simulink model "ALL_JP360_DBW_V6_5_1103"  (R2022a)
settings: Solver=FixedStepAuto  StartTime=0.0  StopTime=inf  FixedStep=0.01  RelTol=1e-3  EnableMultiTasking=on
model workspace (MAT data in the model file):
  g = 9.8
undefined symbols (not defined in the file or in its folder): canChannel, delta_v_p, IPM_Line_C0, IPM_Line_C1, IPM_Line_C2, IPM_Line_C3, M, M_p, MRR_ObjDistX, MRR_ObjDistY, MRR_ObjFusionCamID, MRR_ObjFusionSig, MRR_ObjID, MRR_ObjRelVelX, MRR_ObjRelVelY, MRR_ObjType, MRR_ObjUpdFlg, none, obj_vaild, untracktime, V, videoinput
libraries: canfdmsglib x230, canfdlib x76, slpidlib x24, simulink x18, dspstat3 x14, ctrlSharedLib x1, simulink_extras x1, imaqlib x1, realtime_pacer_lib x1, dspvision x1, visionsinks x1
(part 49 of 55)

== system ALL_JP360_DBW_V6_5_1103/MsgToCAN/CCAN_ADCU_MsgFromCAN/CCAN_ADCU_MRR_0x239 ==
  ACC_BrakePreferred : Inport
  ACC_Status : Inport  Port=2
  ACC_StandstillReq : Inport  Port=3
  ACC_DriveOff : Inport  Port=4
  Bus Creator : BusCreator  Inputs=16  OutDataTypeStr=Bus:CCAN_ADCU_MRR_0x239  NonVirtualBus=on
  Data Type Conversion{1,7,9,12,16} (5 alike) : DataTypeConversion  OutDataTypeStr=int8  SaturateOnIntegerOverflow=off  RndMeth=Floor
  Data Type Conversion{2..6,8,10,13,15} (9 alike) : DataTypeConversion  OutDataTypeStr=boolean  SaturateOnIntegerOverflow=off  RndMeth=Floor
  Data Type Conversion11 : DataTypeConversion  OutDataTypeStr=single  SaturateOnIntegerOverflow=off  RndMeth=Floor
  Data Type Conversion14 : DataTypeConversion  OutDataTypeStr=uint8  SaturateOnIntegerOverflow=off  RndMeth=Floor
  Rolling_Counter : simulink/User-Defined Functions/Rolling_Counter  SystemSampleTime=-1  VariantActivationTime=update diagram  Latency=0  AutoFrameSizeCalculation=off
      settings: SourceProductBaseCode=SL
  CCAN_ADCU_MRR_0x239FromOutData : Outport  OutDataTypeStr=Bus:CCAN_ADCU_MRR_0x239
  wires:
  Data Type Conversion1/1 -> Bus Creator/1  "ABA_Level"
  Data Type Conversion2/1 -> Bus Creator/2  "ABA_Req"
  Data Type Conversion3/1 -> Bus Creator/3  "ABP_Req"
  Data Type Conversion4/1 -> Bus Creator/4  "ACC_BrakePreferred"
  Data Type Conversion5/1 -> Bus Creator/5  "ACC_DriveOff"
  Data Type Conversion6/1 -> Bus Creator/6  "ACC_StandstillReq"
  Data Type Conversion7/1 -> Bus Creator/7  "ACC_Status"
  Data Type Conversion8/1 -> Bus Creator/8  "ACC_VLCMinBrakingReq"
  Data Type Conversion9/1 -> Bus Creator/9  "ACC_VLCShutdownMode"
  Data Type Conversion10/1 -> Bus Creator/10  "AEB_Req"
  Data Type Conversion11/1 -> Bus Creator/11  "AEB_TgtAx"
  Data Type Conversion12/1 -> Bus Creator/12  "AWB_Level"
  Data Type Conversion13/1 -> Bus Creator/13  "AWB_Req"
  Data Type Conversion14/1 -> Bus Creator/14  "Checksum_0x239"
  Data Type Conversion15/1 -> Bus Creator/15  "EBA_Req"
  Data Type Conversion16/1 -> Bus Creator/16  "RollingCounter_0x239"
  Bus Creator/1 -> CCAN_ADCU_MRR_0x239FromOutData/1  "CCAN_ADCU_MRR_0x239FromOutData"
  ACC_BrakePreferred/1 -> Data Type Conversion4/1
  ACC_StandstillReq/1 -> Data Type Conversion6/1
  ACC_Status/1 -> Data Type Conversion7/1
  Rolling_Counter/1 -> Data Type Conversion16/1
  ACC_DriveOff/1 -> Data Type Conversion5/1

== system ALL_JP360_DBW_V6_5_1103/MsgToCAN/CCAN_ADCU_MsgFromCAN/CCAN_ADCU_MRR_0x246 ==
  ACC_Status : Inport
  setvspped : Inport  Port=2
  ACC_TimeGapSet : Inport  Port=3
  ACC_EngineStartstop : Inport  Port=4
  Obj_Speed : Inport  Port=5
  ACC_ObjDetected : Inport  Port=6
  Bus Creator : BusCreator  Inputs=19  OutDataTypeStr=Bus:CCAN_ADCU_MRR_0x246  NonVirtualBus=on
  Constant : Constant  Value=2  OutDataTypeStr=int8
  Constant1 : Constant  Value=2  OutDataTypeStr=int8
  Constant2 : Constant  Value=2  OutDataTypeStr=int8
  Data Type Conversion{1,3,7..10,14..15,19} (9 alike) : DataTypeConversion  OutDataTypeStr=int8  SaturateOnIntegerOverflow=off  RndMeth=Floor
  Data Type Conversion11 : DataTypeConversion  OutDataTypeStr=uint8  SaturateOnIntegerOverflow=off  RndMeth=Floor
  Data Type Conversion{2,4,6,12..13,16..17} (7 alike) : DataTypeConversion  OutDataTypeStr=boolean  SaturateOnIntegerOverflow=off  RndMeth=Floor
  Data Type Conversion18 : DataTypeConversion  OutDataTypeStr=uint8  SaturateOnIntegerOverflow=off  RndMeth=Floor
  Data Type Conversion5 : DataTypeConversion  OutDataTypeStr=single  SaturateOnIntegerOverflow=off  RndMeth=Floor
  Rolling_Counter : simulink/User-Defined Functions/Rolling_Counter  SystemSampleTime=-1  VariantActivationTime=update diagram  Latency=0  AutoFrameSizeCalculation=off
      settings: SourceProductBaseCode=SL
  CCAN_ADCU_MRR_0x246FromOutData : Outport  OutDataTypeStr=Bus:CCAN_ADCU_MRR_0x246
  wires:
  Data Type Conversion1/1 -> Bus Creator/1  "ACC_EngineStartstop"
  Data Type Conversion2/1 -> Bus Creator/2  "ACC_FailInfo"
  Data Type Conversion3/1 -> Bus Creator/3  "ACC_ModeHMI"
  Data Type Conversion4/1 -> Bus Creator/4  "ACC_ObjDetected"
  Data Type Conversion5/1 -> Bus Creator/5  "ACC_SpdSetValue"
  Data Type Conversion6/1 -> Bus Creator/6  "ACC_TakeOverReq"
  Data Type Conversion7/1 -> Bus Creator/7  "ACC_TarObjBarDis"
  Data Type Conversion8/1 -> Bus Creator/8  "ACC_Textinfo"
  Data Type Conversion9/1 -> Bus Creator/9  "ACC_TimeGapSet"
  Data Type Conversion10/1 -> Bus Creator/10  "AEB_Status"
  Data Type Conversion11/1 -> Bus Creator/11  "Checksum_0x246"
  Data Type Conversion12/1 -> Bus Creator/12  "FCW_PedWarningLevel1"
  Data Type Conversion13/1 -> Bus Creator/13  "FCW_PedWarningLevel2"
  Data Type Conversion14/1 -> Bus Creator/14  "FCW_Sensitive"
  Data Type Conversion15/1 -> Bus Creator/15  "FCW_Status"
  Data Type Conversion16/1 -> Bus Creator/16  "FCW_WarningLevel1"
  Data Type Conversion17/1 -> Bus Creator/17  "FCW_WarningLevel2"
  Data Type Conversion18/1 -> Bus Creator/18  "Obj_Speed"
  Data Type Conversion19/1 -> Bus Creator/19  "RollingCounter_0x246"
  Bus Creator/1 -> CCAN_ADCU_MRR_0x246FromOutData/1  "CCAN_ADCU_MRR_0x246FromOutData"
  Rolling_Counter/1 -> Data Type Conversion19/1
  ACC_EngineStartstop/1 -> Data Type Conversion1/1
  ACC_Status/1 -> Data Type Conversion3/1
  setvspped/1 -> Data Type Conversion5/1
  ACC_TimeGapSet/1 -> Data Type Conversion9/1
  Constant/1 -> Data Type Conversion10/1
  Constant1/1 -> Data Type Conversion14/1
  Constant2/1 -> Data Type Conversion15/1
  Obj_Speed/1 -> Data Type Conversion18/1
  ACC_ObjDetected/1 -> Data Type Conversion4/1

== system ALL_JP360_DBW_V6_5_1103/MsgToCAN/CCAN_ADCU_MsgFromCAN/CCAN_ADCU_MRR_FRObj_0x279 ==
  MRR_F_Object_dx : Inport
  MRR_F_Object_dy : Inport  Port=2
  MRR_F_Obj_0x_class : Inport  Port=3
  Bus Creator : BusCreator  Inputs=8  OutDataTypeStr=Bus:CCAN_ADCU_MRR_FRObj_0x279  NonVirtualBus=on
  Data Type Conversion1 : DataTypeConversion  OutDataTypeStr=boolean  SaturateOnIntegerOverflow=off  RndMeth=Floor
  Data Type Conversion2 : DataTypeConversion  OutDataTypeStr=int8  SaturateOnIntegerOverflow=off  RndMeth=Floor
  Data Type Conversion{3..4,6..7} (4 alike) : DataTypeConversion  OutDataTypeStr=single  SaturateOnIntegerOverflow=off  RndMeth=Floor
  Data Type Conversion5 : DataTypeConversion  OutDataTypeStr=int8  SaturateOnIntegerOverflow=off  RndMeth=Floor
  Data Type Conversion8 : DataTypeConversion  OutDataTypeStr=boolean  SaturateOnIntegerOverflow=off  RndMeth=Floor
  CCAN_ADCU_MRR_FRObj_0x279FromOutData : Outport  OutDataTypeStr=Bus:CCAN_ADCU_MRR_FRObj_0x279
  wires:
  Data Type Conversion1/1 -> Bus Creator/1  "MRR_FFTargetDetection"
  Data Type Conversion2/1 -> Bus Creator/2  "MRR_FF_Obj_0x_class"
  Data Type Conversion3/1 -> Bus Creator/3  "MRR_FF_Object_dx"
  Data Type Conversion4/1 -> Bus Creator/4  "MRR_FF_Object_dy"
  Data Type Conversion5/1 -> Bus Creator/5  "MRR_F_Obj_0x_class"
  Data Type Conversion6/1 -> Bus Creator/6  "MRR_F_Object_dx"
  Data Type Conversion7/1 -> Bus Creator/7  "MRR_F_Object_dy"
  Data Type Conversion8/1 -> Bus Creator/8  "MRR_PedDetection"
  Bus Creator/1 -> CCAN_ADCU_MRR_FRObj_0x279FromOutData/1  "CCAN_ADCU_MRR_FRObj_0x279FromOutData"
  MRR_F_Object_dy/1 -> Data Type Conversion7/1
  MRR_F_Object_dx/1 -> Data Type Conversion6/1
  MRR_F_Obj_0x_class/1 -> Data Type Conversion5/1

== system ALL_JP360_DBW_V6_5_1103/MsgToCAN/CCAN_ADCU_MsgFromCAN/CCAN_ADCU_MRR_LRObj_0x480 ==
  MRR_L_Obj_0x_class : Inport
  MRR_L_Object_dx : Inport  Port=2
  MRR_L_Object_dy : Inport  Port=3
  MRR_LeftTargetDetection : Inport  Port=4
  MRR_R_Obj_0x_class : Inport  Port=5
  MRR_R_Object_dx : Inport  Port=6
  MRR_R_Object_dy : Inport  Port=7
  MRR_RightTargetDetection : Inport  Port=8
  Bus Creator : BusCreator  Inputs=8  OutDataTypeStr=Bus:CCAN_ADCU_MRR_LRObj_0x480  NonVirtualBus=on
  Data Type Conversion1 : DataTypeConversion  OutDataTypeStr=int8  SaturateOnIntegerOverflow=off  RndMeth=Floor
  Data Type Conversion{2..3,6..7} (4 alike) : DataTypeConversion  OutDataTypeStr=single  SaturateOnIntegerOverflow=off  RndMeth=Floor
  Data Type Conversion4 : DataTypeConversion  OutDataTypeStr=boolean  SaturateOnIntegerOverflow=off  RndMeth=Floor
  Data Type Conversion5 : DataTypeConversion  OutDataTypeStr=int8  SaturateOnIntegerOverflow=off  RndMeth=Floor
  Data Type Conversion8 : DataTypeConversion  OutDataTypeStr=boolean  SaturateOnIntegerOverflow=off  RndMeth=Floor
  CCAN_ADCU_MRR_LRObj_0x480FromOutData : Outport  OutDataTypeStr=Bus:CCAN_ADCU_MRR_LRObj_0x480
  wires:
  Data Type Conversion1/1 -> Bus Creator/1  "MRR_L_Obj_0x_class"
  Data Type Conversion2/1 -> Bus Creator/2  "MRR_L_Object_dx"
  Data Type Conversion3/1 -> Bus Creator/3  "MRR_L_Object_dy"
  Data Type Conversion4/1 -> Bus Creator/4  "MRR_LeftTargetDetection"
  Data Type Conversion5/1 -> Bus Creator/5  "MRR_R_Obj_0x_class"
  Data Type Conversion6/1 -> Bus Creator/6  "MRR_R_Object_dx"
  Data Type Conversion7/1 -> Bus Creator/7  "MRR_R_Object_dy"
  Data Type Conversion8/1 -> Bus Creator/8  "MRR_RightTargetDetection"
  Bus Creator/1 -> CCAN_ADCU_MRR_LRObj_0x480FromOutData/1  "CCAN_ADCU_MRR_LRObj_0x480FromOutData"
  MRR_L_Obj_0x_class/1 -> Data Type Conversion1/1
  MRR_L_Object_dx/1 -> Data Type Conversion2/1
  MRR_L_Object_dy/1 -> Data Type Conversion3/1
  MRR_LeftTargetDetection/1 -> Data Type Conversion4/1
  MRR_R_Obj_0x_class/1 -> Data Type Conversion5/1
  MRR_R_Object_dx/1 -> Data Type Conversion6/1
  MRR_R_Object_dy/1 -> Data Type Conversion7/1
  MRR_RightTargetDetection/1 -> Data Type Conversion8/1

== system ALL_JP360_DBW_V6_5_1103/MsgToCAN/CCAN_ADCU_MsgFromCAN/CCAN_ADCU_TIMESYNC_analy_620 ==
  Bus Creator : BusCreator  Inputs=6  OutDataTypeStr=Bus:CCAN_ADCU_TIMESYNC_analy_620  NonVirtualBus=on
  Data Type Conversion{1..5} (5 alike) : DataTypeConversion  OutDataTypeStr=int8  SaturateOnIntegerOverflow=off  RndMeth=Floor
  Data Type Conversion6 : DataTypeConversion  OutDataTypeStr=int16  SaturateOnIntegerOverflow=off  RndMeth=Floor
  CCAN_ADCU_TIMESYNC_analy_620FromOutData : Outport  OutDataTypeStr=Bus:CCAN_ADCU_TIMESYNC_analy_620
  wires:
  Data Type Conversion1/1 -> Bus Creator/1  "TIMESYNC_Date"
  Data Type Conversion2/1 -> Bus Creator/2  "TIMESYNC_Hour"
  Data Type Conversion3/1 -> Bus Creator/3  "TIMESYNC_Minute"
  Data Type Conversion4/1 -> Bus Creator/4  "TIMESYNC_Month"
  Data Type Conversion5/1 -> Bus Creator/5  "TIMESYNC_Second"
  Data Type Conversion6/1 -> Bus Creator/6  "TIMESYNC_Year"
  Bus Creator/1 -> CCAN_ADCU_TIMESYNC_analy_620FromOutData/1  "CCAN_ADCU_TIMESYNC_analy_620FromOutData"

== system ALL_JP360_DBW_V6_5_1103/MsgToCAN/CCAN_ADCU_MsgToCAN/CCAN_ADCU_ADCU_0x538 ==
  CCAN_ADCU_ADCU_0x538ToInData : Inport  OutDataTypeStr=Bus:CCAN_ADCU_ADCU_0x538
  CAN FD Pack : canfdmsglib/CAN FD Pack  CANdbFile=HiFire_JPT360_CCAN_Matrix_CAN_V1.72_VP_ADCU.dbc  MsgList=(none)  MsgName=ADCU_0x538  ProtocolMode=CAN FD  MsgIDType=Standard (11-bit identifier)  MsgIdentifier=1336  MsgLength=8  Remote=off  BRSSwitch=on  ApplyMinMax=off  SignalInfo={'ADCU_state','6','2','BE','unsigned','Standard','0','1','0','0','3';'BSD_FCTB_State','0','1','BE','unsigned','Standard','0','1','0','0','1'}
      settings: SourceProductBaseCode=XP,ME,VN  DataFormat=CANdb specified signals
  CAN FD Pack1 : BusSelector  OutputSignals=ADCU_state,BSD_FCTB_State
  CAN_FD_8bit_checksum : simulink/User-Defined Functions/CAN_FD_8bit_checksum  SystemSampleTime=-1  VariantActivationTime=update diagram  Latency=0  AutoFrameSizeCalculation=off
      settings: SourceProductBaseCode=SL
  CCAN_ADCU_ADCU_0x538ToOutData : Outport  OutDataTypeStr=Bus:CAN_FD_MESSAGE_BUS
  wires:
  CCAN_ADCU_ADCU_0x538ToInData/1 -> CAN FD Pack1/1  "CCAN_ADCU_ADCU_0x538ToInData"
  CAN FD Pack/1 -> CAN_FD_8bit_checksum/1  "CCAN_ADCU_ADCU_0x538ToOutData"
  CAN_FD_8bit_checksum/1 -> CCAN_ADCU_ADCU_0x538ToOutData/1  "CCAN_ADCU_ADCU_0x538ToOutData"
  CAN FD Pack1/1 -> CAN FD Pack/1  "<ADCU_state>"
  CAN FD Pack1/2 -> CAN FD Pack/2  "<BSD_FCTB_State>"

== system ALL_JP360_DBW_V6_5_1103/MsgToCAN/CCAN_ADCU_MsgToCAN/CCAN_ADCU_ADCU_CanTSyn_0x570 ==
  CCAN_ADCU_ADCU_CanTSyn_0x570ToInData : Inport  OutDataTypeStr=Bus:CCAN_ADCU_ADCU_CanTSyn_0x570
  CAN FD Pack : canfdmsglib/CAN FD Pack  CANdbFile=HiFire_JPT360_CCAN_Matrix_CAN_V1.72_VP_ADCU.dbc  MsgList=(none)  MsgName=ADCU_CanTSyn_0x570  ProtocolMode=CAN FD  MsgIDType=Standard (11-bit identifier)  MsgIdentifier=1392  MsgLength=8  Remote=off  BRSSwitch=on  ApplyMinMax=off  SignalInfo={'CanTSyn','56','64','BE','unsigned','Standard','0','1','0','0','1.84467440737095e+19'}
      settings: SourceProductBaseCode=XP,ME,VN  DataFormat=CANdb specified signals
  CAN FD Pack1 : BusSelector  OutputSignals=CanTSyn
  CAN_FD_8bit_checksum : simulink/User-Defined Functions/CAN_FD_8bit_checksum  SystemSampleTime=-1  VariantActivationTime=update diagram  Latency=0  AutoFrameSizeCalculation=off
      settings: SourceProductBaseCode=SL
  CCAN_ADCU_ADCU_CanTSyn_0x570ToOutData : Outport  OutDataTypeStr=Bus:CAN_FD_MESSAGE_BUS
  wires:
  CCAN_ADCU_ADCU_CanTSyn_0x570ToInData/1 -> CAN FD Pack1/1  "CCAN_ADCU_ADCU_CanTSyn_0x570ToInData"
  CAN FD Pack/1 -> CAN_FD_8bit_checksum/1  "CCAN_ADCU_ADCU_CanTSyn_0x570ToOutData"
  CAN_FD_8bit_checksum/1 -> CCAN_ADCU_ADCU_CanTSyn_0x570ToOutData/1  "CCAN_ADCU_ADCU_CanTSyn_0x570ToOutData"

== system ALL_JP360_DBW_V6_5_1103/MsgToCAN/CCAN_ADCU_MsgToCAN/CCAN_ADCU_ADCU_DiagResp ==
  CCAN_ADCU_ADCU_DiagRespToInData : Inport  OutDataTypeStr=Bus:CCAN_ADCU_ADCU_DiagResp
  CAN FD Pack : canfdmsglib/CAN FD Pack  CANdbFile=HiFire_JPT360_CCAN_Matrix_CAN_V1.72_VP_ADCU.dbc  MsgList=(none)  MsgName=ADCU_DiagResp  ProtocolMode=CAN FD  MsgIDType=Standard (11-bit identifier)  MsgIdentifier=1817  MsgLength=8  Remote=off  BRSSwitch=on  ApplyMinMax=off  SignalInfo={'DiagRespFromADCU','56','64','BE','unsigned','Standard','0','1','0','0','1.84467440737095e+19'}
      settings: SourceProductBaseCode=XP,ME,VN  DataFormat=CANdb specified signals
  CAN FD Pack1 : BusSelector  OutputSignals=DiagRespFromADCU
  CAN_FD_8bit_checksum : simulink/User-Defined Functions/CAN_FD_8bit_checksum  SystemSampleTime=-1  VariantActivationTime=update diagram  Latency=0  AutoFrameSizeCalculation=off
      settings: SourceProductBaseCode=SL
  CCAN_ADCU_ADCU_DiagRespToOutData : Outport  OutDataTypeStr=Bus:CAN_FD_MESSAGE_BUS
  wires:
  CCAN_ADCU_ADCU_DiagRespToInData/1 -> CAN FD Pack1/1  "CCAN_ADCU_ADCU_DiagRespToInData"
  CAN FD Pack/1 -> CAN_FD_8bit_checksum/1  "CCAN_ADCU_ADCU_DiagRespToOutData"
  CAN_FD_8bit_checksum/1 -> CCAN_ADCU_ADCU_DiagRespToOutData/1  "CCAN_ADCU_ADCU_DiagRespToOutData"

== system ALL_JP360_DBW_V6_5_1103/MsgToCAN/CCAN_ADCU_MsgToCAN/CCAN_ADCU_IPM_0x245 ==
  CCAN_ADCU_IPM_0x245ToInData : Inport  OutDataTypeStr=Bus:CCAN_ADCU_IPM_0x245
  CAN FD Pack : canfdmsglib/CAN FD Pack  CANdbFile=HiFire_JPT360_CCAN_Matrix_CAN_V1.72_VP_ADCU.dbc  MsgList=(none)  MsgName=IPM_0x245  ProtocolMode=CAN FD  MsgIDType=Standard (11-bit identifier)  MsgIdentifier=581  MsgLength=8  Remote=off  BRSSwitch=on  ApplyMinMax=off  SignalInfo={'Checksum_0x245','56','8','BE','unsigned','Standard','0','1','0','0','255';'IPM_ADAS_Alerts','43','3','BE','unsigned','Standard','0','1','0','0','7';'IPM_IHC_HighbeamReq','55','1','BE','unsigned','Standard','0','1','0','0','1';'IPM_IHC_Status','40','3','BE','unsigned','Standard','0','1','0','0','7';'IPM_LDWWarningType','52','2','BE','unsigned','Standard','0','1','0','0','3';'IPM_LaneAssitType','22','3','BE','unsigned','Standard','0','1','0','0','7';'IPM_LaneAssit_HandsonReq','54','1','BE','unsigned','Standard','0','1','0','0','1';'IPM_LaneAssit_LeftVisualization','18','2','BE','unsigned','Standard','0','1','0','0','3';'IPM_LaneAssit_RightVisualization','20','2','BE','unsigned','Standard','0','1','0','0','3';'IPM_LaneAssit_Sensitivity','16','1','BE','unsigned','Standard','0','1','0','0','1';'IPM_LaneAssit_Status','29','3','BE','unsigned','Standard','0','1','0','0','7';'IPM_LaneAssit_TorqueReq','13','11','BE','unsigned','Standard','0','0.01','-10.24','-10.24','10.22';'IPM_LaneAssit_TorqueReqStatus','10','2','BE','unsigned','Standard','0','1','0','0','3';'IPM_LaneAssit_TorqueValidity','12','1','BE','unsigned','Standard','0','1','0','0','1';'IPM_LaneAssit_WarningAudio','17','1','BE','unsigned','Standard','0','1','0','0','1';'IPM_LaneAssit_WarningVibration','9','1','BE','unsigned','Standard','0','1','0','0','1';'IPM_SLA_Spdlimit','32','8','BE','unsigned','Standard','0','1','0','0','255';'IPM_SLA_SpdlimitUnits','24','2','BE','unsigned','Standard','0','1','0','0','3';'IPM_SLA_Status','26','3','BE','unsigned','Standard','0','1','0','0','7';'IPM_TJAICA_Status','47','1','BE','unsigned','Standard','0','1','0','0','1';'RollingCounter_0x245','48','4','BE','unsigned','Standard','0','1','0','0','15'}
      settings: SourceProductBaseCode=XP,ME,VN  DataFormat=CANdb specified signals
  CAN FD Pack1 : BusSelector  OutputSignals=Checksum_0x245,IPM_ADAS_Alerts,IPM_IHC_HighbeamReq,IPM_IHC_Status,IPM_LDWWarningType,IPM_LaneAssitType,IPM_LaneAssit_HandsonReq,IPM_LaneAssit_LeftVisualization,IPM_LaneAssit_RightVisualization,IPM_LaneAssit_Sensitivity,IPM_LaneAssit_Status,IPM_LaneAssit_TorqueReq,IPM_LaneAssit_TorqueReqStatus,IPM_LaneAssit_TorqueValidity,IPM_LaneAssit_WarningAudio,IPM_LaneAssit_WarningVibration,IPM_SLA_Spdlimit,IPM_SLA_SpdlimitUnits,IPM_SLA_Status,IPM_TJAICA_Status,RollingCounter_0x245
  CAN_FD_8bit_checksum : simulink/User-Defined Functions/CAN_FD_8bit_checksum  SystemSampleTime=-1  VariantActivationTime=update diagram  Latency=0  AutoFrameSizeCalculation=off
      settings: SourceProductBaseCode=SL
  CCAN_ADCU_IPM_0x245ToOutData : Outport  OutDataTypeStr=Bus:CAN_FD_MESSAGE_BUS
  wires:
  CCAN_ADCU_IPM_0x245ToInData/1 -> CAN FD Pack1/1  "CCAN_ADCU_IPM_0x245ToInData"
  CAN FD Pack/1 -> CAN_FD_8bit_checksum/1  "CCAN_ADCU_IPM_0x245ToOutData"
  CAN_FD_8bit_checksum/1 -> CCAN_ADCU_IPM_0x245ToOutData/1  "CCAN_ADCU_IPM_0x245ToOutData"
  CAN FD Pack1/1 -> CAN FD Pack/1  "<Checksum_0x245>"
  CAN FD Pack1/2 -> CAN FD Pack/2  "<IPM_ADAS_Alerts>"
  CAN FD Pack1/3 -> CAN FD Pack/3  "<IPM_IHC_HighbeamReq>"
  CAN FD Pack1/4 -> CAN FD Pack/4  "<IPM_IHC_Status>"
  CAN FD Pack1/5 -> CAN FD Pack/5  "<IPM_LDWWarningType>"
  CAN FD Pack1/6 -> CAN FD Pack/6  "<IPM_LaneAssitType>"
  CAN FD Pack1/7 -> CAN FD Pack/7  "<IPM_LaneAssit_HandsonReq>"
  CAN FD Pack1/8 -> CAN FD Pack/8  "<IPM_LaneAssit_LeftVisualization>"
  CAN FD Pack1/9 -> CAN FD Pack/9  "<IPM_LaneAssit_RightVisualization>"
  CAN FD Pack1/10 -> CAN FD Pack/10  "<IPM_LaneAssit_Sensitivity>"
  CAN FD Pack1/11 -> CAN FD Pack/11  "<IPM_LaneAssit_Status>"
  CAN FD Pack1/12 -> CAN FD Pack/12  "<IPM_LaneAssit_TorqueReq>"
  CAN FD Pack1/13 -> CAN FD Pack/13  "<IPM_LaneAssit_TorqueReqStatus>"
  CAN FD Pack1/14 -> CAN FD Pack/14  "<IPM_LaneAssit_TorqueValidity>"
  CAN FD Pack1/15 -> CAN FD Pack/15  "<IPM_LaneAssit_WarningAudio>"
  CAN FD Pack1/16 -> CAN FD Pack/16  "<IPM_LaneAssit_WarningVibration>"
  CAN FD Pack1/17 -> CAN FD Pack/17  "<IPM_SLA_Spdlimit>"
  CAN FD Pack1/18 -> CAN FD Pack/18  "<IPM_SLA_SpdlimitUnits>"
  CAN FD Pack1/19 -> CAN FD Pack/19  "<IPM_SLA_Status>"
  CAN FD Pack1/20 -> CAN FD Pack/20  "<IPM_TJAICA_Status>"
  CAN FD Pack1/21 -> CAN FD Pack/21  "<RollingCounter_0x245>"

== system ALL_JP360_DBW_V6_5_1103/MsgToCAN/CCAN_ADCU_MsgToCAN/CCAN_ADCU_IPM_0x247 ==
  CCAN_ADCU_IPM_0x247ToInData : Inport  OutDataTypeStr=Bus:CCAN_ADCU_IPM_0x247
  CAN FD Pack : canfdmsglib/CAN FD Pack  CANdbFile=HiFire_JPT360_CCAN_Matrix_CAN_V1.72_VP_ADCU.dbc  MsgList=(none)  MsgName=IPM_0x247  ProtocolMode=CAN FD  MsgIDType=Standard (11-bit identifier)  MsgIdentifier=583  MsgLength=8  Remote=off  BRSSwitch=on  ApplyMinMax=off  SignalInfo={'Checksum_0x247','56','8','BE','unsigned','Standard','0','1','0','0','255';'IPM_DCLCSts','5','3','BE','unsigned','Standard','0','1','0','0','7';'IPM_DCLC_manualfeedback','14','4','BE','unsigned','Standard','0','1','0','0','15';'IPM_ELKSts','2','3','BE','unsigned','Standard','0','1','0','0','7';'IPM_Traffic_Sign_Dis','16','8','BE','unsigned','Standard','0','1','0','0','255';'IPM_TurnIndicatorReq','12','2','BE','unsigned','Standard','0','1','0','0','3';'RollingCounter_0x247','48','4','BE','unsigned','Standard','0','1','0','0','15'}
      settings: SourceProductBaseCode=XP,ME,VN  DataFormat=CANdb specified signals
  CAN FD Pack1 : BusSelector  OutputSignals=Checksum_0x247,IPM_DCLCSts,IPM_DCLC_manualfeedback,IPM_ELKSts,IPM_Traffic_Sign_Dis,IPM_TurnIndicatorReq,RollingCounter_0x247
  CAN_FD_8bit_checksum : simulink/User-Defined Functions/CAN_FD_8bit_checksum  SystemSampleTime=-1  VariantActivationTime=update diagram  Latency=0  AutoFrameSizeCalculation=off
      settings: SourceProductBaseCode=SL
  CCAN_ADCU_IPM_0x247ToOutData : Outport  OutDataTypeStr=Bus:CAN_FD_MESSAGE_BUS
  wires:
  CCAN_ADCU_IPM_0x247ToInData/1 -> CAN FD Pack1/1  "CCAN_ADCU_IPM_0x247ToInData"
  CAN FD Pack/1 -> CAN_FD_8bit_checksum/1  "CCAN_ADCU_IPM_0x247ToOutData"
  CAN_FD_8bit_checksum/1 -> CCAN_ADCU_IPM_0x247ToOutData/1  "CCAN_ADCU_IPM_0x247ToOutData"
  CAN FD Pack1/1 -> CAN FD Pack/1  "<Checksum_0x247>"
  CAN FD Pack1/2 -> CAN FD Pack/2  "<IPM_DCLCSts>"
  CAN FD Pack1/3 -> CAN FD Pack/3  "<IPM_DCLC_manualfeedback>"
  CAN FD Pack1/4 -> CAN FD Pack/4  "<IPM_ELKSts>"
  CAN FD Pack1/5 -> CAN FD Pack/5  "<IPM_Traffic_Sign_Dis>"
  CAN FD Pack1/6 -> CAN FD Pack/6  "<IPM_TurnIndicatorReq>"
  CAN FD Pack1/7 -> CAN FD Pack/7  "<RollingCounter_0x247>"

== system ALL_JP360_DBW_V6_5_1103/MsgToCAN/CCAN_ADCU_MsgToCAN/CCAN_ADCU_IPM_LeftLine_0x278 ==
  CCAN_ADCU_IPM_LeftLine_0x278ToInData : Inport  OutDataTypeStr=Bus:CCAN_ADCU_IPM_LeftLine_0x278
  CAN FD Pack : canfdmsglib/CAN FD Pack  CANdbFile=HiFire_JPT360_CCAN_Matrix_CAN_V1.72_VP_ADCU.dbc  MsgList=(none)  MsgName=IPM_LeftLine_0x278  ProtocolMode=CAN FD  MsgIDType=Standard (11-bit identifier)  MsgIdentifier=632  MsgLength=8  Remote=off  BRSSwitch=on  ApplyMinMax=off  SignalInfo={'IPM_LedtLine_dx_start','0','8','BE','unsigned','Standard','0','0.25','0','0','63.75';'IPM_LeftLine_dx_lookhead','27','9','BE','unsigned','Standard','0','0.25','0','0','127.75';'IPM_LeftLine_dy','20','12','BE','unsigned','Standard','0','0.0039062','-8','-8','7.9961';'IPM_LeftLine_hor_curvature_alteration','58','10','BE','unsigned','Standard','0','0.0001','-0.015','-0.015','0.0873';'IPM_LeftLine_hor_curve','33','10','BE','unsigned','Standard','0','0.0001','-0.015','-0.015','0.0873';'IPM_LeftLine_yawangle','52','12','BE','unsigned','Standard','0','0.00048828','-1','-1','0.99951'}
      settings: SourceProductBaseCode=XP,ME,VN  DataFormat=CANdb specified signals
  CAN FD Pack1 : BusSelector  OutputSignals=IPM_LedtLine_dx_start,IPM_LeftLine_dx_lookhead,IPM_LeftLine_dy,IPM_LeftLine_hor_curvature_alteration,IPM_LeftLine_hor_curve,IPM_LeftLine_yawangle
  CCAN_ADCU_IPM_LeftLine_0x278ToOutData : Outport  OutDataTypeStr=Bus:CAN_FD_MESSAGE_BUS
  wires:
  CCAN_ADCU_IPM_LeftLine_0x278ToInData/1 -> CAN FD Pack1/1  "CCAN_ADCU_IPM_LeftLine_0x278ToInData"
  CAN FD Pack/1 -> CCAN_ADCU_IPM_LeftLine_0x278ToOutData/1  "CCAN_ADCU_IPM_LeftLine_0x278ToOutData"
  CAN FD Pack1/1 -> CAN FD Pack/1  "<IPM_LedtLine_dx_start>"
  CAN FD Pack1/2 -> CAN FD Pack/2  "<IPM_LeftLine_dx_lookhead>"
  CAN FD Pack1/3 -> CAN FD Pack/3  "<IPM_LeftLine_dy>"
  CAN FD Pack1/4 -> CAN FD Pack/4  "<IPM_LeftLine_hor_curvature_alteration>"
  CAN FD Pack1/5 -> CAN FD Pack/5  "<IPM_LeftLine_hor_curve>"
  CAN FD Pack1/6 -> CAN FD Pack/6  "<IPM_LeftLine_yawangle>"

== system ALL_JP360_DBW_V6_5_1103/MsgToCAN/CCAN_ADCU_MsgToCAN/CCAN_ADCU_IPM_LeftLine_0x280 ==
  CCAN_ADCU_IPM_LeftLine_0x280ToInData : Inport  OutDataTypeStr=Bus:CCAN_ADCU_IPM_LeftLine_0x280
  CAN FD Pack : canfdmsglib/CAN FD Pack  CANdbFile=HiFire_JPT360_CCAN_Matrix_CAN_V1.72_VP_ADCU.dbc  MsgList=(none)  MsgName=IPM_LeftLine_0x280  ProtocolMode=CAN FD  MsgIDType=Standard (11-bit identifier)  MsgIdentifier=640  MsgLength=8  Remote=off  BRSSwitch=on  ApplyMinMax=off  SignalInfo={'IPM_LaneAssit_LeftLeftVisualization','0','2','BE','unsigned','Standard','0','1','0','0','3';'IPM_LeftLeftLine_Color','13','3','BE','unsigned','Standard','0','1','0','0','7';'IPM_LeftLeftLine_Type','10','3','BE','unsigned','Standard','0','1','0','0','7';'IPM_LeftLeftLine_curvature_alteration','56','12','BE','unsigned','Standard','0','0.0001','-0.015','-0.015','0.0873';'IPM_LeftLeftLine_dy','28','12','BE','unsigned','Standard','0','0.0039062','-8','-8','7.9961';'IPM_LeftLeftLine_hor_curve','33','10','BE','unsigned','Standard','0','0.0001','-0.015','-0.015','0.0873';'IPM_LeftLeftLine_yawangle','52','12','BE','unsigned','Standard','0','0.00048828','-1','-1','0.99951';'IPM_LeftLine_Color','5','3','BE','unsigned','Standard','0','1','0','0','7';'IPM_LeftLine_Type','2','3','BE','unsigned','Standard','0','1','0','0','7'}
      settings: SourceProductBaseCode=XP,ME,VN  DataFormat=CANdb specified signals
  CAN FD Pack1 : BusSelector  OutputSignals=IPM_LaneAssit_LeftLeftVisualization,IPM_LeftLeftLine_Color,IPM_LeftLeftLine_Type,IPM_LeftLeftLine_curvature_alteration,IPM_LeftLeftLine_dy,IPM_LeftLeftLine_hor_curve,IPM_LeftLeftLine_yawangle,IPM_LeftLine_Color,IPM_LeftLine_Type
  CCAN_ADCU_IPM_LeftLine_0x280ToOutData : Outport  OutDataTypeStr=Bus:CAN_FD_MESSAGE_BUS
  wires:
  CCAN_ADCU_IPM_LeftLine_0x280ToInData/1 -> CAN FD Pack1/1  "CCAN_ADCU_IPM_LeftLine_0x280ToInData"
  CAN FD Pack/1 -> CCAN_ADCU_IPM_LeftLine_0x280ToOutData/1  "CCAN_ADCU_IPM_LeftLine_0x280ToOutData"
  CAN FD Pack1/1 -> CAN FD Pack/1  "<IPM_LaneAssit_LeftLeftVisualization>"
  CAN FD Pack1/2 -> CAN FD Pack/2  "<IPM_LeftLeftLine_Color>"
  CAN FD Pack1/3 -> CAN FD Pack/3  "<IPM_LeftLeftLine_Type>"
  CAN FD Pack1/4 -> CAN FD Pack/4  "<IPM_LeftLeftLine_curvature_alteration>"
  CAN FD Pack1/5 -> CAN FD Pack/5  "<IPM_LeftLeftLine_dy>"
  CAN FD Pack1/6 -> CAN FD Pack/6  "<IPM_LeftLeftLine_hor_curve>"
  CAN FD Pack1/7 -> CAN FD Pack/7  "<IPM_LeftLeftLine_yawangle>"
  CAN FD Pack1/8 -> CAN FD Pack/8  "<IPM_LeftLine_Color>"
  CAN FD Pack1/9 -> CAN FD Pack/9  "<IPM_LeftLine_Type>"

== system ALL_JP360_DBW_V6_5_1103/MsgToCAN/CCAN_ADCU_MsgToCAN/CCAN_ADCU_IPM_RightLine_0x490 ==
  CCAN_ADCU_IPM_RightLine_0x490ToInData : Inport  OutDataTypeStr=Bus:CCAN_ADCU_IPM_RightLine_0x490
  CAN FD Pack : canfdmsglib/CAN FD Pack  CANdbFile=HiFire_JPT360_CCAN_Matrix_CAN_V1.72_VP_ADCU.dbc  MsgList=(none)  MsgName=IPM_RightLine_0x490  ProtocolMode=CAN FD  MsgIDType=Standard (11-bit identifier)  MsgIdentifier=1168  MsgLength=8  Remote=off  BRSSwitch=on  ApplyMinMax=off  SignalInfo={'IPM_RightLine_dx_lookhead','27','9','BE','unsigned','Standard','0','0.25','0','0','127.75';'IPM_RightLine_dx_start','0','8','BE','unsigned','Standard','0','0.25','0','0','63.75';'IPM_RightLine_dy','20','12','BE','unsigned','Standard','0','0.0039062','-8','-8','7.9961';'IPM_RightLine_hor_curvature_alteration','58','10','BE','unsigned','Standard','0','0.0001','-0.015','-0.015','0.0873';'IPM_RightLine_hor_curve','33','10','BE','unsigned','Standard','0','0.0001','-0.015','-0.015','0.0873';'IPM_RightLine_yawangle','52','12','BE','unsigned','Standard','0','0.00048828','-1','-1','0.99951'}
      settings: SourceProductBaseCode=XP,ME,VN  DataFormat=CANdb specified signals
  CAN FD Pack1 : BusSelector  OutputSignals=IPM_RightLine_dx_lookhead,IPM_RightLine_dx_start,IPM_RightLine_dy,IPM_RightLine_hor_curvature_alteration,IPM_RightLine_hor_curve,IPM_RightLine_yawangle
  CCAN_ADCU_IPM_RightLine_0x490ToOutData : Outport  OutDataTypeStr=Bus:CAN_FD_MESSAGE_BUS
  wires:
  CCAN_ADCU_IPM_RightLine_0x490ToInData/1 -> CAN FD Pack1/1  "CCAN_ADCU_IPM_RightLine_0x490ToInData"
  CAN FD Pack/1 -> CCAN_ADCU_IPM_RightLine_0x490ToOutData/1  "CCAN_ADCU_IPM_RightLine_0x490ToOutData"
  CAN FD Pack1/1 -> CAN FD Pack/1  "<IPM_RightLine_dx_lookhead>"
  CAN FD Pack1/2 -> CAN FD Pack/2  "<IPM_RightLine_dx_start>"
  CAN FD Pack1/3 -> CAN FD Pack/3  "<IPM_RightLine_dy>"
  CAN FD Pack1/4 -> CAN FD Pack/4  "<IPM_RightLine_hor_curvature_alteration>"
  CAN FD Pack1/5 -> CAN FD Pack/5  "<IPM_RightLine_hor_curve>"
  CAN FD Pack1/6 -> CAN FD Pack/6  "<IPM_RightLine_yawangle>"

== system ALL_JP360_DBW_V6_5_1103/MsgToCAN/CCAN_ADCU_MsgToCAN/CCAN_ADCU_IPM_RightLine_0x491 ==
  CCAN_ADCU_IPM_RightLine_0x491ToInData : Inport  OutDataTypeStr=Bus:CCAN_ADCU_IPM_RightLine_0x491
  CAN FD Pack : canfdmsglib/CAN FD Pack  CANdbFile=HiFire_JPT360_CCAN_Matrix_CAN_V1.72_VP_ADCU.dbc  MsgList=(none)  MsgName=IPM_RightLine_0x491  ProtocolMode=CAN FD  MsgIDType=Standard (11-bit identifier)  MsgIdentifier=1169  MsgLength=8  Remote=off  BRSSwitch=on  ApplyMinMax=off  SignalInfo={'IPM_LaneAssit_RightRightVisualization','0','2','BE','unsigned','Standard','0','1','0','0','3';'IPM_RighRightLine_Color','13','3','BE','unsigned','Standard','0','1','0','0','7';'IPM_RightLine_Color','5','3','BE','unsigned','Standard','0','1','0','0','7';'IPM_RightLine_Type','2','3','BE','unsigned','Standard','0','1','0','0','7';'IPM_RightRighLine_Type','10','3','BE','unsigned','Standard','0','1','0','0','7';'IPM_RightRightLine_curvature_alteration','56','12','BE','unsigned','Standard','0','0.0001','-0.015','-0.015','0.0873';'IPM_RightRightLine_dy','28','12','BE','unsigned','Standard','0','0.0039062','-8','-8','7.9961';'IPM_RightRightLine_hor_curve','33','10','BE','unsigned','Standard','0','0.0001','-0.015','-0.015','0.0873';'IPM_RightRightLine_yawangle','52','12','BE','unsigned','Standard','0','0.00048828','-1','-1','0.99951'}
      settings: SourceProductBaseCode=XP,ME,VN  DataFormat=CANdb specified signals
  CAN FD Pack1 : BusSelector  OutputSignals=IPM_LaneAssit_RightRightVisualization,IPM_RighRightLine_Color,IPM_RightLine_Color,IPM_RightLine_Type,IPM_RightRighLine_Type,IPM_RightRightLine_curvature_alteration,IPM_RightRightLine_dy,IPM_RightRightLine_hor_curve,IPM_RightRightLine_yawangle
  CCAN_ADCU_IPM_RightLine_0x491ToOutData : Outport  OutDataTypeStr=Bus:CAN_FD_MESSAGE_BUS
  wires:
  CCAN_ADCU_IPM_RightLine_0x491ToInData/1 -> CAN FD Pack1/1  "CCAN_ADCU_IPM_RightLine_0x491ToInData"
  CAN FD Pack/1 -> CCAN_ADCU_IPM_RightLine_0x491ToOutData/1  "CCAN_ADCU_IPM_RightLine_0x491ToOutData"
  CAN FD Pack1/1 -> CAN FD Pack/1  "<IPM_LaneAssit_RightRightVisualization>"
  CAN FD Pack1/2 -> CAN FD Pack/2  "<IPM_RighRightLine_Color>"
  CAN FD Pack1/3 -> CAN FD Pack/3  "<IPM_RightLine_Color>"
  CAN FD Pack1/4 -> CAN FD Pack/4  "<IPM_RightLine_Type>"
  CAN FD Pack1/5 -> CAN FD Pack/5  "<IPM_RightRighLine_Type>"
  CAN FD Pack1/6 -> CAN FD Pack/6  "<IPM_RightRightLine_curvature_alteration>"
  CAN FD Pack1/7 -> CAN FD Pack/7  "<IPM_RightRightLine_dy>"
  CAN FD Pack1/8 -> CAN FD Pack/8  "<IPM_RightRightLine_hor_curve>"
  CAN FD Pack1/9 -> CAN FD Pack/9  "<IPM_RightRightLine_yawangle>"

== system ALL_JP360_DBW_V6_5_1103/MsgToCAN/CCAN_ADCU_MsgToCAN/CCAN_ADCU_IPM_VLC_0x293 ==
  CCAN_ADCU_IPM_VLC_0x293ToInData : Inport  OutDataTypeStr=Bus:CCAN_ADCU_IPM_VLC_0x293
  CAN FD Pack : canfdmsglib/CAN FD Pack  CANdbFile=HiFire_JPT360_CCAN_Matrix_CAN_V1.72_VP_ADCU.dbc  MsgList=(none)  MsgName=IPM_VLC_0x293  ProtocolMode=CAN FD  MsgIDType=Standard (11-bit identifier)  MsgIdentifier=659  MsgLength=8  Remote=off  BRSSwitch=on  ApplyMinMax=off  SignalInfo={'ACC_Torque_Request','16','16','BE','unsigned','Standard','0','0.5','-15000','-15000','15000';'ACC_Torque_Request_Status','7','1','BE','unsigned','Standard','0','1','0','0','1';'Checksum_0x293','56','8','BE','unsigned','Standard','0','1','0','0','255';'RollingCounter_0x293','48','4','BE','unsigned','Standard','0','1','0','0','15'}
      settings: SourceProductBaseCode=XP,ME,VN  DataFormat=CANdb specified signals
  CAN FD Pack1 : BusSelector  OutputSignals=ACC_Torque_Request,ACC_Torque_Request_Status,Checksum_0x293,RollingCounter_0x293
  CAN_FD_8bit_checksum : simulink/User-Defined Functions/CAN_FD_8bit_checksum  SystemSampleTime=-1  VariantActivationTime=update diagram  Latency=0  AutoFrameSizeCalculation=off
      settings: SourceProductBaseCode=SL
  CCAN_ADCU_IPM_VLC_0x293ToOutData : Outport  OutDataTypeStr=Bus:CAN_FD_MESSAGE_BUS
  wires:
  CCAN_ADCU_IPM_VLC_0x293ToInData/1 -> CAN FD Pack1/1  "CCAN_ADCU_IPM_VLC_0x293ToInData"
  CAN FD Pack/1 -> CAN_FD_8bit_checksum/1  "CCAN_ADCU_IPM_VLC_0x293ToOutData"
  CAN_FD_8bit_checksum/1 -> CCAN_ADCU_IPM_VLC_0x293ToOutData/1  "CCAN_ADCU_IPM_VLC_0x293ToOutData"
  CAN FD Pack1/1 -> CAN FD Pack/1  "<ACC_Torque_Request>"
  CAN FD Pack1/2 -> CAN FD Pack/2  "<ACC_Torque_Request_Status>"
  CAN FD Pack1/3 -> CAN FD Pack/3  "<Checksum_0x293>"
  CAN FD Pack1/4 -> CAN FD Pack/4  "<RollingCounter_0x293>"

== system ALL_JP360_DBW_V6_5_1103/MsgToCAN/CCAN_ADCU_MsgToCAN/CCAN_ADCU_MRR_0x238 ==
  CCAN_ADCU_MRR_0x238ToInData : Inport  OutDataTypeStr=Bus:CCAN_ADCU_MRR_0x238
  CAN FD Pack : canfdmsglib/CAN FD Pack  CANdbFile=HiFire_JPT360_CCAN_Matrix_CAN_V1.72_VP_ADCU.dbc  MsgList=(none)  MsgName=MRR_0x238  ProtocolMode=CAN FD  MsgIDType=Standard (11-bit identifier)  MsgIdentifier=568  MsgLength=8  Remote=off  BRSSwitch=on  ApplyMinMax=off  SignalInfo={'ACC_TgtAx','53','11','BE','unsigned','Standard','0','0.05','-5','-5','7.75';'ACC_TgtAxLowerComftBand','8','8','BE','unsigned','Standard','0','0.05','0','0','3.2';'ACC_TgtAxLowerLim','24','8','BE','unsigned','Standard','0','0.1','-12.7','-12.7','0';'ACC_TgtAxUpperComftBand','0','8','BE','unsigned','Standard','0','0.05','0','0','3.2';'ACC_TgtAxUpperLim','16','8','BE','unsigned','Standard','0','0.1','0','0','12.7';'Checksum_0x238','56','8','BE','unsigned','Standard','0','1','0','0','255';'RollingCounter_0x238','48','4','BE','unsigned','Standard','0','1','0','0','15'}
      settings: SourceProductBaseCode=XP,ME,VN  DataFormat=CANdb specified signals
  CAN FD Pack1 : BusSelector  OutputSignals=ACC_TgtAx,ACC_TgtAxLowerComftBand,ACC_TgtAxLowerLim,ACC_TgtAxUpperComftBand,ACC_TgtAxUpperLim,Checksum_0x238,RollingCounter_0x238
  CAN_FD_8bit_checksum : simulink/User-Defined Functions/CAN_FD_8bit_checksum  SystemSampleTime=-1  VariantActivationTime=update diagram  Latency=0  AutoFrameSizeCalculation=off
      settings: SourceProductBaseCode=SL
  CCAN_ADCU_MRR_0x238ToOutData : Outport  OutDataTypeStr=Bus:CAN_FD_MESSAGE_BUS
  wires:
  CCAN_ADCU_MRR_0x238ToInData/1 -> CAN FD Pack1/1  "CCAN_ADCU_MRR_0x238ToInData"
  CAN FD Pack/1 -> CAN_FD_8bit_checksum/1  "CCAN_ADCU_MRR_0x238ToOutData"
  CAN_FD_8bit_checksum/1 -> CCAN_ADCU_MRR_0x238ToOutData/1  "CCAN_ADCU_MRR_0x238ToOutData"
  CAN FD Pack1/1 -> CAN FD Pack/1  "<ACC_TgtAx>"
  CAN FD Pack1/2 -> CAN FD Pack/2  "<ACC_TgtAxLowerComftBand>"
  CAN FD Pack1/3 -> CAN FD Pack/3  "<ACC_TgtAxLowerLim>"
  CAN FD Pack1/4 -> CAN FD Pack/4  "<ACC_TgtAxUpperComftBand>"
  CAN FD Pack1/5 -> CAN FD Pack/5  "<ACC_TgtAxUpperLim>"
  CAN FD Pack1/6 -> CAN FD Pack/6  "<Checksum_0x238>"
  CAN FD Pack1/7 -> CAN FD Pack/7  "<RollingCounter_0x238>"

== system ALL_JP360_DBW_V6_5_1103/MsgToCAN/CCAN_ADCU_MsgToCAN/CCAN_ADCU_MRR_0x239 ==
  CCAN_ADCU_MRR_0x239ToInData : Inport  OutDataTypeStr=Bus:CCAN_ADCU_MRR_0x239
  CAN FD Pack : canfdmsglib/CAN FD Pack  CANdbFile=HiFire_JPT360_CCAN_Matrix_CAN_V1.72_VP_ADCU.dbc  MsgList=(none)  MsgName=MRR_0x239  ProtocolMode=CAN FD  MsgIDType=Standard (11-bit identifier)  MsgIdentifier=569  MsgLength=8  Remote=off  BRSSwitch=on  ApplyMinMax=off  SignalInfo={'ABA_Level','8','2','BE','unsigned','Standard','0','1','0','0','3';'ABA_Req','23','1','BE','unsigned','Standard','0','1','0','0','1';'ABP_Req','21','1','BE','unsigned','Standard','0','1','0','0','1';'ACC_BrakePreferred','1','1','BE','unsigned','Standard','0','1','0','0','1';'ACC_DriveOff','15','1','BE','unsigned','Standard','0','1','0','0','1';'ACC_StandstillReq','14','1','BE','unsigned','Standard','0','1','0','0','1';'ACC_Status','3','3','BE','unsigned','Standard','0','1','0','0','7';'ACC_VLCMinBrakingReq','0','1','BE','unsigned','Standard','0','1','0','0','1';'ACC_VLCShutdownMode','6','2','BE','unsigned','Standard','0','1','0','0','3';'AEB_Req','13','1','BE','unsigned','Standard','0','1','0','0','1';'AEB_TgtAx','32','16','BE','unsigned','Standard','0','0.05','-16','-16','16';'AWB_Level','16','4','BE','unsigned','Standard','0','1','0','0','15';'AWB_Req','22','1','BE','unsigned','Standard','0','1','0','0','1';'Checksum_0x239','56','8','BE','unsigned','Standard','0','1','0','0','255';'EBA_Req','12','1','BE','unsigned','Standard','0','1','0','0','1';'RollingCounter_0x239','48','4','BE','unsigned','Standard','0','1','0','0','15'}
      settings: SourceProductBaseCode=XP,ME,VN  DataFormat=CANdb specified signals
  CAN FD Pack1 : BusSelector  OutputSignals=ABA_Level,ABA_Req,ABP_Req,ACC_BrakePreferred,ACC_DriveOff,ACC_StandstillReq,ACC_Status,ACC_VLCMinBrakingReq,ACC_VLCShutdownMode,AEB_Req,AEB_TgtAx,AWB_Level,AWB_Req,Checksum_0x239,EBA_Req,RollingCounter_0x239
  CAN_FD_8bit_checksum : simulink/User-Defined Functions/CAN_FD_8bit_checksum  SystemSampleTime=-1  VariantActivationTime=update diagram  Latency=0  AutoFrameSizeCalculation=off
      settings: SourceProductBaseCode=SL
  CCAN_ADCU_MRR_0x239ToOutData : Outport  OutDataTypeStr=Bus:CAN_FD_MESSAGE_BUS
  wires:
  CCAN_ADCU_MRR_0x239ToInData/1 -> CAN FD Pack1/1  "CCAN_ADCU_MRR_0x239ToInData"
  CAN FD Pack/1 -> CAN_FD_8bit_checksum/1  "CCAN_ADCU_MRR_0x239ToOutData"
  CAN_FD_8bit_checksum/1 -> CCAN_ADCU_MRR_0x239ToOutData/1  "CCAN_ADCU_MRR_0x239ToOutData"
  CAN FD Pack1/1 -> CAN FD Pack/1  "<ABA_Level>"
  CAN FD Pack1/2 -> CAN FD Pack/2  "<ABA_Req>"
  CAN FD Pack1/3 -> CAN FD Pack/3  "<ABP_Req>"
  CAN FD Pack1/4 -> CAN FD Pack/4  "<ACC_BrakePreferred>"
  CAN FD Pack1/5 -> CAN FD Pack/5  "<ACC_DriveOff>"
  CAN FD Pack1/6 -> CAN FD Pack/6  "<ACC_StandstillReq>"
  CAN FD Pack1/7 -> CAN FD Pack/7  "<ACC_Status>"
  CAN FD Pack1/8 -> CAN FD Pack/8  "<ACC_VLCMinBrakingReq>"
  CAN FD Pack1/9 -> CAN FD Pack/9  "<ACC_VLCShutdownMode>"
  CAN FD Pack1/10 -> CAN FD Pack/10  "<AEB_Req>"
  CAN FD Pack1/11 -> CAN FD Pack/11  "<AEB_TgtAx>"
  CAN FD Pack1/12 -> CAN FD Pack/12  "<AWB_Level>"
  CAN FD Pack1/13 -> CAN FD Pack/13  "<AWB_Req>"
  CAN FD Pack1/14 -> CAN FD Pack/14  "<Checksum_0x239>"
  CAN FD Pack1/15 -> CAN FD Pack/15  "<EBA_Req>"
  CAN FD Pack1/16 -> CAN FD Pack/16  "<RollingCounter_0x239>"

== system ALL_JP360_DBW_V6_5_1103/MsgToCAN/CCAN_ADCU_MsgToCAN/CCAN_ADCU_MRR_0x246 ==
  CCAN_ADCU_MRR_0x246ToInData : Inport  OutDataTypeStr=Bus:CCAN_ADCU_MRR_0x246
  CAN FD Pack : canfdmsglib/CAN FD Pack  CANdbFile=HiFire_JPT360_CCAN_Matrix_CAN_V1.72_VP_ADCU.dbc  MsgList=(none)  MsgName=MRR_0x246  ProtocolMode=CAN FD  MsgIDType=Standard (11-bit identifier)  MsgIdentifier=582  MsgLength=8  Remote=off  BRSSwitch=on  ApplyMinMax=off  SignalInfo={'ACC_EngineStartstop','28','2','BE','unsigned','Standard','0','1','0','0','3';'ACC_FailInfo','19','1','BE','unsigned','Standard','0','1','0','0','1';'ACC_ModeHMI','16','3','BE','unsigned','Standard','0','1','0','0','7';'ACC_ObjDetected','8','1','BE','unsigned','Standard','0','1','0','0','1';'ACC_SpdSetValue','15','9','BE','unsigned','Standard','0','0.5','0','0','255.5';'ACC_TakeOverReq','20','1','BE','unsigned','Standard','0','1','0','0','1';'ACC_TarObjBarDis','12','3','BE','unsigned','Standard','0','1','0','0','7';'ACC_Textinfo','52','6','BE','unsigned','Standard','0','1','0','0','63';'ACC_TimeGapSet','9','3','BE','unsigned','Standard','0','1','0','0','7';'AEB_Status','25','3','BE','unsigned','Standard','0','1','0','0','7';'Checksum_0x246','56','8','BE','unsigned','Standard','0','1','0','0','255';'FCW_PedWarningLevel1','21','1','BE','unsigned','Standard','0','1','0','0','1';'FCW_PedWarningLevel2','24','1','BE','unsigned','Standard','0','1','0','0','1';'FCW_Sensitive','22','2','BE','unsigned','Standard','0','1','0','0','3';'FCW_Status','37','3','BE','unsigned','Standard','0','1','0','0','7';'FCW_WarningLevel1','31','1','BE','unsigned','Standard','0','1','0','0','1';'FCW_WarningLevel2','30','1','BE','unsigned','Standard','0','1','0','0','1';'Obj_Speed','42','8','BE','unsigned','Standard','0','1','0','0','255';'RollingCounter_0x246','48','4','BE','unsigned','Standard','0','1','0','0','15'}
      settings: SourceProductBaseCode=XP,ME,VN  DataFormat=CANdb specified signals
  CAN FD Pack1 : BusSelector  OutputSignals=ACC_EngineStartstop,ACC_FailInfo,ACC_ModeHMI,ACC_ObjDetected,ACC_SpdSetValue,ACC_TakeOverReq,ACC_TarObjBarDis,ACC_Textinfo,ACC_TimeGapSet,AEB_Status,Checksum_0x246,FCW_PedWarningLevel1,FCW_PedWarningLevel2,FCW_Sensitive,FCW_Status,FCW_WarningLevel1,FCW_WarningLevel2,Obj_Speed,RollingCounter_0x246
  CAN_FD_8bit_checksum : simulink/User-Defined Functions/CAN_FD_8bit_checksum  SystemSampleTime=-1  VariantActivationTime=update diagram  Latency=0  AutoFrameSizeCalculation=off
      settings: SourceProductBaseCode=SL
  CCAN_ADCU_MRR_0x246ToOutData : Outport  OutDataTypeStr=Bus:CAN_FD_MESSAGE_BUS
  wires:
  CCAN_ADCU_MRR_0x246ToInData/1 -> CAN FD Pack1/1  "CCAN_ADCU_MRR_0x246ToInData"
  CAN FD Pack/1 -> CAN_FD_8bit_checksum/1  "CCAN_ADCU_MRR_0x246ToOutData"
  CAN_FD_8bit_checksum/1 -> CCAN_ADCU_MRR_0x246ToOutData/1  "CCAN_ADCU_MRR_0x246ToOutData"
  CAN FD Pack1/1 -> CAN FD Pack/1  "<ACC_EngineStartstop>"
  CAN FD Pack1/2 -> CAN FD Pack/2  "<ACC_FailInfo>"
  CAN FD Pack1/3 -> CAN FD Pack/3  "<ACC_ModeHMI>"
  CAN FD Pack1/4 -> CAN FD Pack/4  "<ACC_ObjDetected>"
  CAN FD Pack1/5 -> CAN FD Pack/5  "<ACC_SpdSetValue>"
  CAN FD Pack1/6 -> CAN FD Pack/6  "<ACC_TakeOverReq>"
  CAN FD Pack1/7 -> CAN FD Pack/7  "<ACC_TarObjBarDis>"
  CAN FD Pack1/8 -> CAN FD Pack/8  "<ACC_Textinfo>"
  CAN FD Pack1/9 -> CAN FD Pack/9  "<ACC_TimeGapSet>"
  CAN FD Pack1/10 -> CAN FD Pack/10  "<AEB_Status>"
  CAN FD Pack1/11 -> CAN FD Pack/11  "<Checksum_0x246>"
  CAN FD Pack1/12 -> CAN FD Pack/12  "<FCW_PedWarningLevel1>"
  CAN FD Pack1/13 -> CAN FD Pack/13  "<FCW_PedWarningLevel2>"
  CAN FD Pack1/14 -> CAN FD Pack/14  "<FCW_Sensitive>"
  CAN FD Pack1/15 -> CAN FD Pack/15  "<FCW_Status>"
  CAN FD Pack1/16 -> CAN FD Pack/16  "<FCW_WarningLevel1>"
  CAN FD Pack1/17 -> CAN FD Pack/17  "<FCW_WarningLevel2>"
  CAN FD Pack1/18 -> CAN FD Pack/18  "<Obj_Speed>"
  CAN FD Pack1/19 -> CAN FD Pack/19  "<RollingCounter_0x246>"

== system ALL_JP360_DBW_V6_5_1103/MsgToCAN/CCAN_ADCU_MsgToCAN/CCAN_ADCU_MRR_FRObj_0x279 ==
  CCAN_ADCU_MRR_FRObj_0x279ToInData : Inport  OutDataTypeStr=Bus:CCAN_ADCU_MRR_FRObj_0x279
  CAN FD Pack : canfdmsglib/CAN FD Pack  CANdbFile=HiFire_JPT360_CCAN_Matrix_CAN_V1.72_VP_ADCU.dbc  MsgList=(none)  MsgName=MRR_FRObj_0x279  ProtocolMode=CAN FD  MsgIDType=Standard (11-bit identifier)  MsgIdentifier=633  MsgLength=8  Remote=off  BRSSwitch=on  ApplyMinMax=off  SignalInfo={'MRR_FFTargetDetection','54','1','BE','unsigned','Standard','0','1','0','0','1';'MRR_FF_Obj_0x_class','40','3','BE','unsigned','Standard','0','1','0','0','7';'MRR_FF_Object_dx','36','12','BE','unsigned','Standard','0','0.0625','0','0','255.875';'MRR_FF_Object_dy','43','9','BE','unsigned','Standard','0','0.0625','-15','-15','15';'MRR_F_Obj_0x_class','16','3','BE','unsigned','Standard','0','1','0','0','7';'MRR_F_Object_dx','12','12','BE','unsigned','Standard','0','0.0625','0','0','255.875';'MRR_F_Object_dy','19','9','BE','unsigned','Standard','0','0.0625','-15','-15','15';'MRR_PedDetection','55','1','BE','unsigned','Standard','0','1','0','0','1'}
      settings: SourceProductBaseCode=XP,ME,VN  DataFormat=CANdb specified signals
  CAN FD Pack1 : BusSelector  OutputSignals=MRR_FFTargetDetection,MRR_FF_Obj_0x_class,MRR_FF_Object_dx,MRR_FF_Object_dy,MRR_F_Obj_0x_class,MRR_F_Object_dx,MRR_F_Object_dy,MRR_PedDetection
  CAN_FD_8bit_checksum : simulink/User-Defined Functions/CAN_FD_8bit_checksum  SystemSampleTime=-1  VariantActivationTime=update diagram  Latency=0  AutoFrameSizeCalculation=off
      settings: SourceProductBaseCode=SL
  CCAN_ADCU_MRR_FRObj_0x279ToOutData : Outport  OutDataTypeStr=Bus:CAN_FD_MESSAGE_BUS
  wires:
  CCAN_ADCU_MRR_FRObj_0x279ToInData/1 -> CAN FD Pack1/1  "CCAN_ADCU_MRR_FRObj_0x279ToInData"
  CAN FD Pack/1 -> CAN_FD_8bit_checksum/1  "CCAN_ADCU_MRR_FRObj_0x279ToOutData"
  CAN_FD_8bit_checksum/1 -> CCAN_ADCU_MRR_FRObj_0x279ToOutData/1  "CCAN_ADCU_MRR_FRObj_0x279ToOutData"
  CAN FD Pack1/1 -> CAN FD Pack/1  "<MRR_FFTargetDetection>"
  CAN FD Pack1/2 -> CAN FD Pack/2  "<MRR_FF_Obj_0x_class>"
  CAN FD Pack1/3 -> CAN FD Pack/3  "<MRR_FF_Object_dx>"
  CAN FD Pack1/4 -> CAN FD Pack/4  "<MRR_FF_Object_dy>"
  CAN FD Pack1/5 -> CAN FD Pack/5  "<MRR_F_Obj_0x_class>"
  CAN FD Pack1/6 -> CAN FD Pack/6  "<MRR_F_Object_dx>"
  CAN FD Pack1/7 -> CAN FD Pack/7  "<MRR_F_Object_dy>"
  CAN FD Pack1/8 -> CAN FD Pack/8  "<MRR_PedDetection>"

== system ALL_JP360_DBW_V6_5_1103/MsgToCAN/CCAN_ADCU_MsgToCAN/CCAN_ADCU_MRR_LRObj_0x480 ==
  CCAN_ADCU_MRR_LRObj_0x480ToInData : Inport  OutDataTypeStr=Bus:CCAN_ADCU_MRR_LRObj_0x480
  CAN FD Pack : canfdmsglib/CAN FD Pack  CANdbFile=HiFire_JPT360_CCAN_Matrix_CAN_V1.72_VP_ADCU.dbc  MsgList=(none)  MsgName=MRR_LRObj_0x480  ProtocolMode=CAN FD  MsgIDType=Standard (11-bit identifier)  MsgIdentifier=1152  MsgLength=8  Remote=off  BRSSwitch=on  ApplyMinMax=off  SignalInfo={'MRR_L_Obj_0x_class','16','3','BE','unsigned','Standard','0','1','0','0','7';'MRR_L_Object_dx','12','12','BE','unsigned','Standard','0','0.0625','0','0','255.875';'MRR_L_Object_dy','19','9','BE','unsigned','Standard','0','0.0625','-15','-15','15';'MRR_LeftTargetDetection','54','1','BE','unsigned','Standard','0','1','0','0','1';'MRR_R_Obj_0x_class','40','3','BE','unsigned','Standard','0','1','0','0','7';'MRR_R_Object_dx','36','12','BE','unsigned','Standard','0','0.0625','0','0','255.875';'MRR_R_Object_dy','43','9','BE','unsigned','Standard','0','0.0625','-15','-15','15';'MRR_RightTargetDetection','55','1','BE','unsigned','Standard','0','1','0','0','1'}
      settings: SourceProductBaseCode=XP,ME,VN  DataFormat=CANdb specified signals
  CAN FD Pack1 : BusSelector  OutputSignals=MRR_L_Obj_0x_class,MRR_L_Object_dx,MRR_L_Object_dy,MRR_LeftTargetDetection,MRR_R_Obj_0x_class,MRR_R_Object_dx,MRR_R_Object_dy,MRR_RightTargetDetection
  CAN_FD_8bit_checksum : simulink/User-Defined Functions/CAN_FD_8bit_checksum  SystemSampleTime=-1  VariantActivationTime=update diagram  Latency=0  AutoFrameSizeCalculation=off
      settings: SourceProductBaseCode=SL
  CCAN_ADCU_MRR_LRObj_0x480ToOutData : Outport  OutDataTypeStr=Bus:CAN_FD_MESSAGE_BUS
  wires:
  CCAN_ADCU_MRR_LRObj_0x480ToInData/1 -> CAN FD Pack1/1  "CCAN_ADCU_MRR_LRObj_0x480ToInData"
  CAN FD Pack/1 -> CAN_FD_8bit_checksum/1  "CCAN_ADCU_MRR_LRObj_0x480ToOutData"
  CAN_FD_8bit_checksum/1 -> CCAN_ADCU_MRR_LRObj_0x480ToOutData/1  "CCAN_ADCU_MRR_LRObj_0x480ToOutData"
  CAN FD Pack1/1 -> CAN FD Pack/1  "<MRR_L_Obj_0x_class>"
  CAN FD Pack1/2 -> CAN FD Pack/2  "<MRR_L_Object_dx>"
  CAN FD Pack1/3 -> CAN FD Pack/3  "<MRR_L_Object_dy>"
  CAN FD Pack1/4 -> CAN FD Pack/4  "<MRR_LeftTargetDetection>"
  CAN FD Pack1/5 -> CAN FD Pack/5  "<MRR_R_Obj_0x_class>"
  CAN FD Pack1/6 -> CAN FD Pack/6  "<MRR_R_Object_dx>"
  CAN FD Pack1/7 -> CAN FD Pack/7  "<MRR_R_Object_dy>"
  CAN FD Pack1/8 -> CAN FD Pack/8  "<MRR_RightTargetDetection>"

== system ALL_JP360_DBW_V6_5_1103/MsgToCAN/CCAN_ADCU_MsgToCAN/CCAN_ADCU_TIMESYNC_analy_620 ==
  CCAN_ADCU_TIMESYNC_analy_620ToInData : Inport  OutDataTypeStr=Bus:CCAN_ADCU_TIMESYNC_analy_620
  CAN FD Pack : canfdmsglib/CAN FD Pack  CANdbFile=HiFire_JPT360_CCAN_Matrix_CAN_V1.72_VP_ADCU.dbc  MsgList=(none)  MsgName=TIMESYNC_analy_620  ProtocolMode=CAN FD  MsgIDType=Standard (11-bit identifier)  MsgIdentifier=1568  MsgLength=8  Remote=off  BRSSwitch=on  ApplyMinMax=off  SignalInfo={'TIMESYNC_Date','16','8','BE','unsigned','Standard','0','1','1','1','31';'TIMESYNC_Hour','24','8','BE','unsigned','Standard','0','1','0','0','23';'TIMESYNC_Minute','32','8','BE','unsigned','Standard','0','1','0','0','59';'TIMESYNC_Month','8','8','BE','unsigned','Standard','0','1','1','1','12';'TIMESYNC_Second','40','8','BE','unsigned','Standard','0','1','0','0','59';'TIMESYNC_Year','0','8','BE','unsigned','Standard','0','1','2017','2017','2272'}
      settings: SourceProductBaseCode=XP,ME,VN  DataFormat=CANdb specified signals
  CAN FD Pack1 : BusSelector  OutputSignals=TIMESYNC_Date,TIMESYNC_Hour,TIMESYNC_Minute,TIMESYNC_Month,TIMESYNC_Second,TIMESYNC_Year
  CAN_FD_8bit_checksum : simulink/User-Defined Functions/CAN_FD_8bit_checksum  SystemSampleTime=-1  VariantActivationTime=update diagram  Latency=0  AutoFrameSizeCalculation=off
      settings: SourceProductBaseCode=SL
  CCAN_ADCU_TIMESYNC_analy_620ToOutData : Outport  OutDataTypeStr=Bus:CAN_FD_MESSAGE_BUS
  wires:
  CCAN_ADCU_TIMESYNC_analy_620ToInData/1 -> CAN FD Pack1/1  "CCAN_ADCU_TIMESYNC_analy_620ToInData"
  CAN FD Pack/1 -> CAN_FD_8bit_checksum/1  "CCAN_ADCU_TIMESYNC_analy_620ToOutData"
  CAN_FD_8bit_checksum/1 -> CCAN_ADCU_TIMESYNC_analy_620ToOutData/1  "CCAN_ADCU_TIMESYNC_analy_620ToOutData"
  CAN FD Pack1/1 -> CAN FD Pack/1  "<TIMESYNC_Date>"
  CAN FD Pack1/2 -> CAN FD Pack/2  "<TIMESYNC_Hour>"
  CAN FD Pack1/3 -> CAN FD Pack/3  "<TIMESYNC_Minute>"
  CAN FD Pack1/4 -> CAN FD Pack/4  "<TIMESYNC_Month>"
  CAN FD Pack1/5 -> CAN FD Pack/5  "<TIMESYNC_Second>"
  CAN FD Pack1/6 -> CAN FD Pack/6  "<TIMESYNC_Year>"
